simulink subsystem "MPC10_nlpsol"  (R2022b)
settings: Solver=VariableStepAuto  StartTime=0.0  StopTime=10.0  RelTol=1e-3
undefined symbols (not defined in the file): param_jointspace_ct, param_MPC10, param_robot, param_traj_data, param_weight_init
settings Model: Creator=emu  LastModifiedBy=emu
settings OptimizationCC: ReuseModelBlockBuffer=on

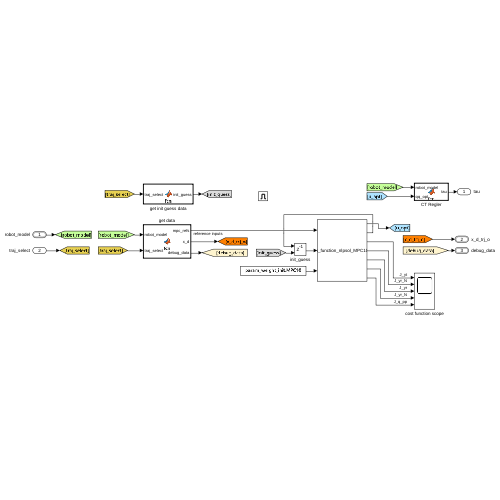
[thumbnail: Simulink's stored preview of the top-level diagram]
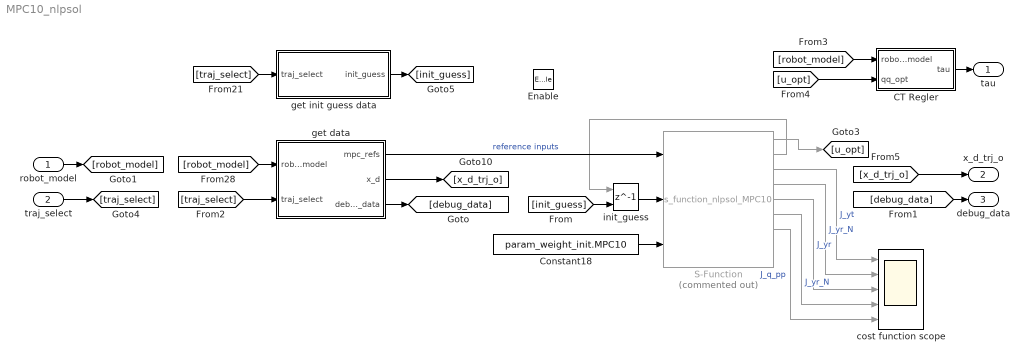
== system MPC10_nlpsol ==
  robot_model : Inport  OutDataTypeStr=Bus: robot_model
  traj_select : Inport  Port=2
  Enable : EnablePort
  CT Regler : MATLAB Function  TreatAsAtomicUnit=on
  Constant18 : Constant  Value=param_weight_init.MPC10  VectorParams1D=off
  S-Function : S-Function  Commented=on  FunctionName=s_function_nlpsol_MPC10  Parameters='s_functions/ur5e_6dof/MPC10.casadi', 'MPC10'  SFunctionModules='MPC10'  SFunctionDeploymentMode=off  EnableBusSupport=off
  cost function scope : Scope  NumInputPorts=5
  get data : MATLAB Function  TreatAsAtomicUnit=on
  get init guess data : MATLAB Function  TreatAsAtomicUnit=on
  init_guess : Delay  DelayLength=1  InitialConditionSource=Input port  InitialCondition=1
      settings: InputPortMap=u0,p4
  tau : Outport
  x_d_trj_o : Outport  Port=2  OutDataTypeStr=Bus: x_d
  debug_data : Outport  Port=3  OutDataTypeStr=Bus: debug_data_bus
  wires:
  S-Function/2 -> init_guess/1
  S-Function/7 -> cost function scope/5  "J_q_pp"
  [debug_data] -> debug_data/1
  get data/1(mpc_refs) -> S-Function/1  "reference inputs"
  [robot_model] -> get data/1(robot_model)
  get data/2(x_d) -> [x_d_trj_o]
  [traj_select] -> get init guess data/1(traj_select)
  [init_guess] -> init_guess/2
  CT Regler/1(tau) -> tau/1
  S-Function/6 -> cost function scope/4  "J_yr_N"
  traj_select/1 -> [traj_select]
  [u_opt] -> CT Regler/2(qq_opt)
  S-Function/4 -> cost function scope/2  "J_yr_N"
  [traj_select] -> get data/2(traj_select)
  [robot_model] -> CT Regler/1(robot_model)
  robot_model/1 -> [robot_model]
  init_guess/1 -> S-Function/2
  get init guess data/1(init_guess) -> [init_guess]
  get data/3(debug_data) -> [debug_data]
  Constant18/1 -> S-Function/3
  S-Function/3 -> cost function scope/1  "J_yt"
  S-Function/5 -> cost function scope/3  "J_yr"
  [x_d_trj_o] -> x_d_trj_o/1
  S-Function/1 -> [u_opt]

== matlab function MPC10_nlpsol/CT Regler ==
  data: robot_model input Bus: robot_model; tau output; qq_opt input; param_robot parameter; param_jointspace_ct parameter
function tau = fcn(robot_model, qq_opt, param_robot, param_jointspace_ct)

n = param_robot.n_DOF;

if size(qq_opt, 2) ~= 0 && size(qq_opt, 1) ~= 1
    q = robot_model.q;      % generalized coordinates
    q_p = robot_model.q_p;  % time derivative of generalized coordinates
    
    q_d = qq_opt(1:n);
    q_d_p = qq_opt(n+1:2*n);
    q_d_pp = qq_opt(2*n+1:end);
    
    M = robot_model.M;      % inertia matrix
    C_rnea = robot_model.C_rnea; % C_rnea(q, q_p) = C(q, q_p)q_p + g(q) = n(q, q_p)
    
    e = q - q_d;
    e_p = q_p - q_d_p;
    
    K_D_q = param_jointspace_ct.MPC10.K_D_q;
    K_P_q = param_jointspace_ct.MPC10.K_P_q;
    tau = M*(q_d_pp - K_D_q * e_p - K_P_q * e) + C_rnea;
else
    tau = zeros(n,1);
end

== matlab function MPC10_nlpsol/get data ==
  settings: updateMethod=DISCRETE  sampleTime=param_global.Ta
  data: mpc_refs output; robot_model input Bus: robot_model; param_MPC10 parameter; x_d output Bus: x_d; debug_data output Bus: debug_data_bus; param_traj_data parameter; traj_select input
function [mpc_refs, x_d, debug_data] = fcn(robot_model, param_MPC10, param_traj_data, traj_select)
persistent cnt;

if(isempty(cnt))
    cnt = 1;
end

param_MPC = param_MPC10;
N         = param_MPC.N;
N_step    = param_MPC.N_step;

% Parameters
q    = robot_model.q;      % generalized coordinates
q_p  = robot_model.q_p;  % time derivative of generalized coordinates
q_pp = robot_model.q_pp;
H    = robot_model.H;
J    = robot_model.J;
J_p  = robot_model.J_p;

R = H(1:3,1:3);% desired Orientation as rotational matrix
R_d = param_traj_data.R_d(:,:, cnt, traj_select);
q_d = param_traj_data.q_d(:, cnt, traj_select);

%y_q_err = quat_mult(y_q_e, quat_inv(param_traj_data.q_d(1:4, cnt, traj_select)));
q_err = rotm2quat_v4(R*R_d');
%y_q_e = rotm2quat_v4(R);
q_e = quat_mult(q_d, q_err);

% Current Pose of Endeffector
y = [H(1:3,4); q_e];
y_p = J*q_p;
y_pp = J*q_pp + J_p*q_p;



x_k = [q;q_p];

% Assemble vector of recieved output measurements
p_d    = param_traj_data.p_d(   1:3, cnt : N_step : cnt + (N)*N_step, traj_select);
%p_d_p  = param_traj_data.p_d_p( 1:3, cnt : N_step : cnt + (N)*N_step, traj_select);
%p_d_pp = param_traj_data.p_d_pp(1:3, cnt : N_step : cnt + (N)*N_step, traj_select);

% RPY XYZ angles
%Phi_d = param_traj_data.Phi_d(      1:3, cnt : N_step : cnt + (N) * N_step, traj_select ); % (Phi_0 ... Phi_N)
%Phi_d_p = param_traj_data.Phi_d_p(  1:3, cnt : N_step : cnt + (N) * N_step, traj_select ); % (Phi_p_0 ... Phi_p_N)
%Phi_d_pp = param_traj_data.Phi_d_pp(1:3, cnt : N_step : cnt + (N) * N_step, traj_select ); % (Phi_pp_0 ... Phi_pp_N)

q_d    = param_traj_data.q_d(      1:4, cnt : N_step : cnt + (N)*N_step, traj_select);
%q_d_p  = param_traj_data.q_d_p(    1:4, cnt : N_step : cnt + (N)*N_step, traj_select);
%q_d_pp = param_traj_data.q_d_pp(   1:4, cnt : N_step : cnt + (N)*N_step, traj_select);

omega_d   = param_traj_data.omega_d(  1:3, cnt : N_step : cnt + (N)*N_step, traj_select);
omega_d_p = param_traj_data.omega_d_p(1:3, cnt : N_step : cnt + (N)*N_step, traj_select);

alpha_d    = param_traj_data.alpha_d(           :, cnt : N_step : cnt + (N)*N_step, traj_select);
alpha_d_p  = param_traj_data.alpha_d_p(         :, cnt : N_step : cnt + (N)*N_step, traj_select);
alpha_d_pp = param_traj_data.alpha_d_pp(        :, cnt : N_step : cnt + (N)*N_step, traj_select);
rot_ax_d   = param_traj_data.rot_ax_d(          :, cnt : N_step : cnt + (N)*N_step, traj_select);
alpha_d_offset = param_traj_data.alpha_d_offset(:, cnt : N_step : cnt + (N)*N_step, traj_select);
q_d_rel = param_traj_data.q_d_rel(              :, cnt : N_step : cnt + (N)*N_step, traj_select);

diff_variant_mode = struct;
diff_variant_mode.numdiff = 1; % default forward, central, backward deviation
diff_variant_mode.savgol = 2; % savgol filtering and deviation
diff_variant_mode.savgol_v2 = 3; % savgol filtering without additional equations and deviation
diff_variant_mode.numdiff_twotimes = 4; % forward, central, backward deviation with two different time steps

diff_variant = diff_variant_mode.numdiff;

y_d = [p_d; q_d];
%y_d_p = [p_d_p; omega_d];
%y_d_pp = [p_d_pp; omega_d_p];

%% Reference out
p_d_kp1 = param_traj_data.p_d(   1:3, cnt+1, traj_select);
q_d_kp1 = param_traj_data.q_d(   1:4, cnt+1, traj_select);

if(diff_variant == diff_variant_mode.numdiff_twotimes)
    if(N_step == 1)
        y_d = [p_d; q_d];
    else
        y_d    = [[p_d(:,1), p_d_kp1, p_d(:,2:end-1)]; [q_d(:,1), q_d_kp1, q_d(:,2:end-1)]];
    end
    mpc_refs = [x_k(:); y_d(:)];
else
    y_d_kp1 = [p_d_kp1;  q_d_kp1];
    p_d_kp2 = param_traj_data.p_d(   1:3, cnt+2, traj_select);
    q_d_kp2 = param_traj_data.q_d(   1:4, cnt+2, traj_select);
    y_d_kp2 = [p_d_kp2;  q_d_kp2];
    mpc_refs = [x_k(:); y_d(:); y_d_kp1(:); y_d_kp2(:)];
end

%% TRAJECTORY OUT
x_d.p_d       = param_traj_data.p_d(1:3, cnt , traj_select);    %y0
x_d.p_d_p     = param_traj_data.p_d_p(1:3, cnt , traj_select);  %y0p
x_d.p_d_pp    = param_traj_data.p_d_pp(1:3, cnt , traj_select); %y0pp
x_d.Phi_d     = param_traj_data.Phi_d(:, cnt , traj_select);
x_d.Phi_d_p   = param_traj_data.Phi_d_p(:, cnt, traj_select);
x_d.Phi_d_pp  = param_traj_data.Phi_d_pp(:,cnt, traj_select);
x_d.R_d       = R_d;
x_d.q_d       = q_d(1:4, 1);
x_d.q_d_p     = param_traj_data.q_d_p(1:4, cnt, traj_select);
x_d.q_d_pp    = param_traj_data.q_d_pp(1:4, cnt, traj_select);
x_d.omega_d   = omega_d(1:3, 1);
x_d.omega_d_p = omega_d_p(1:3, 1);
x_d.alpha_d    = alpha_d(:, 1);
x_d.alpha_d_p  = alpha_d_p(:, 1);
x_d.alpha_d_pp = alpha_d_pp(:, 1);
x_d.rot_ax_d   = rot_ax_d(:, 1);
x_d.alpha_d_offset = alpha_d_offset(:, 1);
x_d.q_d_rel = q_d_rel(:, 1);

%% DEBUG
debug_data.p           = y(1:3);
debug_data.p_p         = y_p(1:3);
debug_data.p_pp        = y_pp(1:3);
debug_data.Phi     = rotm2eul_v2(R);
debug_data.Phi_p   = [0; 0; 0]; % ?????? Phi_p = T * omega?
debug_data.Phi_pp  = [0; 0; 0]; % ??????
debug_data.q           = y(4:7);
debug_data.omega       = y_p(4:6);
debug_data.omega_p     = y_pp(4:6);
debug_data.p_err       = y(1:3) - param_traj_data.p_d(:, cnt, traj_select);
debug_data.p_p_err     = y_p(1:3) - param_traj_data.p_d_p(:, cnt, traj_select);
debug_data.p_pp_err    = y_pp(1:3) - param_traj_data.p_d_pp(:, cnt, traj_select);
debug_data.q_err       = q_err;
debug_data.omega_err   = y_p(4:6)  - omega_d(1:3, 1);
debug_data.omega_p_err = y_pp(4:6) - omega_d_p(1:3, 1);

cnt = cnt+1;

== matlab function MPC10_nlpsol/get init guess data ==
  data: traj_select input; param_MPC10_init_guess parameter; init_guess output
function init_guess   = fcn(traj_select, param_MPC10_init_guess)

%init_guess = param_MPC10_init_guess.init_guess(1,:);
init_guess = param_MPC10_init_guess.init_guess(traj_select,:);
